simulink model "CT_SigmaDelta"  (Simulink 7.9)
settings: Solver=ode45  StartTime=0.0  StopTime=1  RelTol=1e-6
PreLoadFcn:
  | load one_stage.mat
libraries: dspmlti4 x7, simulink x2
(part 1 of 5)
settings Model: Creator=abehbood  LastModifiedBy=Arnaldi Isacco  CovSaveName=MOD  CovHTMLOptions=-sRT=1 -aTS=1 -bRG=1 -bTC=1 -hTR=0 -nFC=0 -scm=1 -bcm=1 -xEv=0  CovCumulativeVarName=MOD1
settings Model: CovPath=|
  | Averaging
  | Power Spectral
  | Density
settings SolverCC: ConsecutiveZCsStepRelTol=128*eps  ZeroCrossControl=DisableAll
settings DataIOCC: LimitDataPoints=off  SaveFormat=StructureWithTime  SaveOutput=off  SignalLogging=off  DSMLogging=off  SaveTime=off
settings OptimizationCC: InitFltsAndDblsToZero=on
settings DebuggingCC: AlgebraicLoopMsg=none  SaveWithParameterizedLinksMsg=none  SignalResolutionControl=TryResolveAllWithWarning  FcnCallInpInsideContextMsg=Use local settings  StrictBusMsg=Warning
settings SFSimCC: SimParseCustomCode=off
settings RTWCC: GenerateMakefile=off
settings GRTTargetCC: TargetFcnLib=ansi_tfl_tmw.mat  CombineOutputUpdateFcns=off  GRTInterface=on
settings ConfigurationSet: Description=SimMechanics 2G

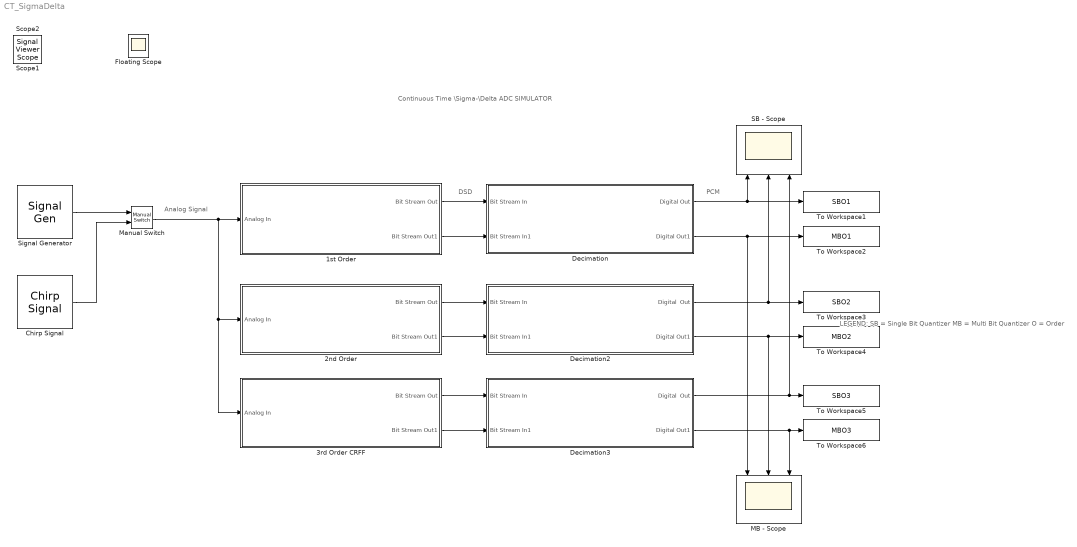
== system CT_SigmaDelta ==
  note: Continuous Time
      | \Sigma-\Delta ADC
      | SIMULATOR
  note: Analog Signal
  note: LEGEND:
      |
      | SB = Single Bit Quantizer
      |
      | MB = Multi Bit Quantizer
      |
      | O = Order
  note: DSD
  note: PCM
  1st Order : Subsystem
  "2nd Order  " : Subsystem
  3rd Order CRFF : Subsystem
  Chirp Signal : simulink/Sources/Chirp Signal  f1=0.1  T=24/24  f2=10000
  Decimation : Subsystem
  Decimation2 : Subsystem
  Decimation3 : Subsystem
  MB - Scope : Scope  NumInputPorts=3
      settings: ShowLegends=on  TimeRange=0.008  YMin=-1.25~-1.25~-1.25  YMax=1.25~1.25~1.25  SaveName=ScopeData2
  Manual Switch : simulink/Signal Routing/Manual Switch  sw=1  action=0  varsize=off
  SB - Scope : Scope  NumInputPorts=3
      settings: ShowLegends=on  TimeRange=0.008  YMin=-1.25~-1.25~-0.75  YMax=1.25~1.25~0.75
  Signal Generator : SignalGenerator  Frequency=6283  Units=rad/sec
  To Workspace1 : ToWorkspace  VariableName=SBO1  SampleTime=-1
  To Workspace2 : ToWorkspace  VariableName=MBO1  SampleTime=-1
  To Workspace3 : ToWorkspace  VariableName=SBO2  SampleTime=-1
  To Workspace4 : ToWorkspace  VariableName=MBO2  SampleTime=-1
  To Workspace5 : ToWorkspace  VariableName=SBO3  SampleTime=-1
  To Workspace6 : ToWorkspace  VariableName=MBO3  SampleTime=-1
  Floating Scope : Scope
      settings: Floating=on  YMin=-1  YMax=1
  Scope1 : SignalViewerScope  IOType=viewer  RefreshTime=0.035000
  Scope2 : SignalViewerScope  IOType=viewer  RefreshTime=0.035000
  wires:
  Decimation/1(Digital Out) -> SB - Scope/1, To Workspace1/1
  Decimation/2(Digital Out1) -> MB - Scope/1, To Workspace2/1
  Decimation2/1(Digital  Out) -> SB - Scope/2, To Workspace3/1
  Decimation2/2(Digital Out1) -> MB - Scope/2, To Workspace4/1
  Decimation3/1(Digital  Out) -> To Workspace5/1, SB - Scope/3
  Decimation3/2(Digital Out1) -> To Workspace6/1, MB - Scope/3
  1st Order/1(Bit Stream Out) -> Decimation/1(Bit Stream In)
  "2nd Order  "/1(Bit Stream Out) -> Decimation2/1(Bit Stream In)
  "2nd Order  "/2(Bit Stream Out1) -> Decimation2/2(Bit Stream In1)
  3rd Order CRFF/1(Bit Stream Out) -> Decimation3/1(Bit Stream In)
  3rd Order CRFF/2(Bit Stream Out1) -> Decimation3/2(Bit Stream In1)
  Signal Generator/1 -> Manual Switch/1
  Manual Switch/1 -> 1st Order/1("Analog In "), "2nd Order  "/1(Analog In), 3rd Order CRFF/1(Analog In)
  Chirp Signal/1 -> Manual Switch/2
  1st Order/2(Bit Stream Out1) -> Decimation/2(Bit Stream In1)

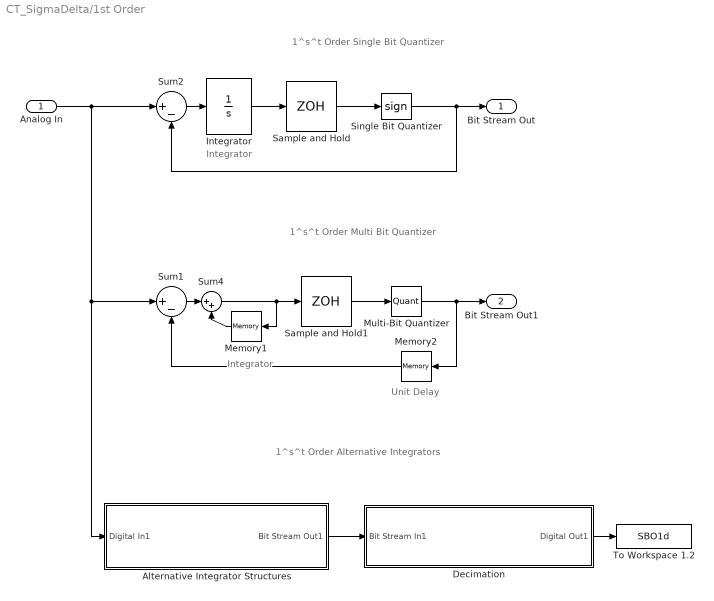
== system CT_SigmaDelta/1st Order ==
  note: 1^s^t Order Single Bit Quantizer
  note: 1^s^t Order Multi Bit Quantizer
  note: Integrator
  note: 1^s^t Order Alternative Integrators
  note: Unit Delay
  note: Integrator
  "Analog In " : Inport
  Alternative Integrator Structures : Subsystem
  Decimation : Subsystem
  Integrator : Integrator
  Memory1 : Memory  InheritSampleTime=on  LinearizeAsDelay=on
  Memory2 : Memory  InheritSampleTime=on  LinearizeAsDelay=on
  Multi-Bit Quantizer : Quantizer  QuantizationInterval=0.14  SampleTime=1/(48e3*64)
  Sample and Hold : ZeroOrderHold  SampleTime=1/(48e3*64)
  Sample and Hold1 : ZeroOrderHold  SampleTime=1/(48e3*64)
  Single Bit Quantizer : Signum  SampleTime=1/(48e3*64)
  Sum1 : Sum  Inputs=|+-  AccumDataTypeStr=double  SampleTime=1/(48e3*64)
  Sum2 : Sum  Inputs=|+-  AccumDataTypeStr=double  SampleTime=1/(48e3*64)
  Sum4 : Sum  Inputs=|++
  To Workspace 1.2 : ToWorkspace  VariableName=SBO1d  SampleTime=-1
  Bit Stream Out : Outport  OutDataTypeStr=double
  Bit Stream Out1 : Outport  Port=2  OutDataTypeStr=double
  wires:
  "Analog In "/1 -> Sum2/1, Sum1/1, Alternative Integrator Structures/1(Digital In1)
  Integrator/1 -> Sample and Hold/1
  Sum2/1 -> Integrator/1
  Sample and Hold/1 -> Single Bit Quantizer/1
  Single Bit Quantizer/1 -> Bit Stream Out/1, Sum2/2
  Alternative Integrator Structures/1(Bit Stream Out1) -> Decimation/1(Bit Stream In1)
  Decimation/1(Digital Out1) -> To Workspace 1.2/1
  Memory1/1 -> Sum4/2
  Sum4/1 -> Memory1/1, Sample and Hold1/1
  Sum1/1 -> Sum4/1
  Sample and Hold1/1 -> Multi-Bit Quantizer/1
  Multi-Bit Quantizer/1 -> Memory2/1, Bit Stream Out1/1
  Memory2/1 -> Sum1/2

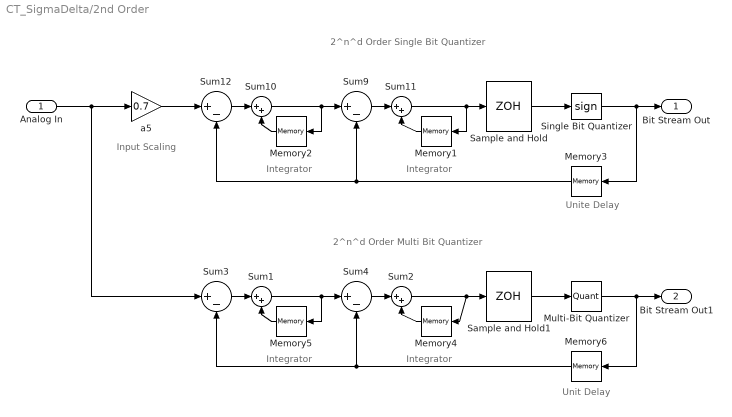
== system CT_SigmaDelta/2nd Order   ==
  note: 2^n^d Order Single Bit Quantizer
  note: 2^n^d Order Multi Bit Quantizer
  note: Input Scaling
  note: Integrator
  note: Integrator
  note: Integrator
  note: Integrator
  note: Unite Delay
  note: Unit Delay
  Analog In : Inport
  Memory{1..6} (6 alike) : Memory  InheritSampleTime=on  LinearizeAsDelay=on
  Multi-Bit Quantizer : Quantizer  QuantizationInterval=0.15  SampleTime=1/(48e3*64)
  Sample and Hold : ZeroOrderHold  SampleTime=1/(48e3*64)
  Sample and Hold1 : ZeroOrderHold  SampleTime=1/(48e3*64)
  Single Bit Quantizer : Signum  SampleTime=1/(48e3*64)
  Sum{1..2,10..11} (4 alike) : Sum  Inputs=|++  SampleTime=1/(48e3*64)
  Sum{3..4,9,12} (4 alike) : Sum  Inputs=|+-  AccumDataTypeStr=double  SampleTime=1/(48e3*64)
  a5 : Gain  Gain=0.7  SampleTime=1/(48e3*64)
  Bit Stream Out : Outport  OutDataTypeStr=double
  Bit Stream Out1 : Outport  Port=2  OutDataTypeStr=double
  wires:
  Analog In/1 -> a5/1, Sum3/1
  Sample and Hold/1 -> Single Bit Quantizer/1
  Sum9/1 -> Sum11/1
  Sum12/1 -> Sum10/1
  Single Bit Quantizer/1 -> Bit Stream Out/1, Memory3/1
  a5/1 -> Sum12/1
  Sample and Hold1/1 -> Multi-Bit Quantizer/1
  Sum4/1 -> Sum2/1
  Sum3/1 -> Sum1/1
  Multi-Bit Quantizer/1 -> Bit Stream Out1/1, Memory6/1
  Sum1/1 -> Sum4/1, Memory5/1
  Memory5/1 -> Sum1/2
  Sum10/1 -> Memory2/1, Sum9/1
  Memory2/1 -> Sum10/2
  Memory1/1 -> Sum11/2
  Sum11/1 -> Sample and Hold/1, Memory1/1
  Memory4/1 -> Sum2/2
  Sum2/1 -> Sample and Hold1/1, Memory4/1
  Memory3/1 -> Sum12/2, Sum9/2
  Memory6/1 -> Sum3/2, Sum4/2

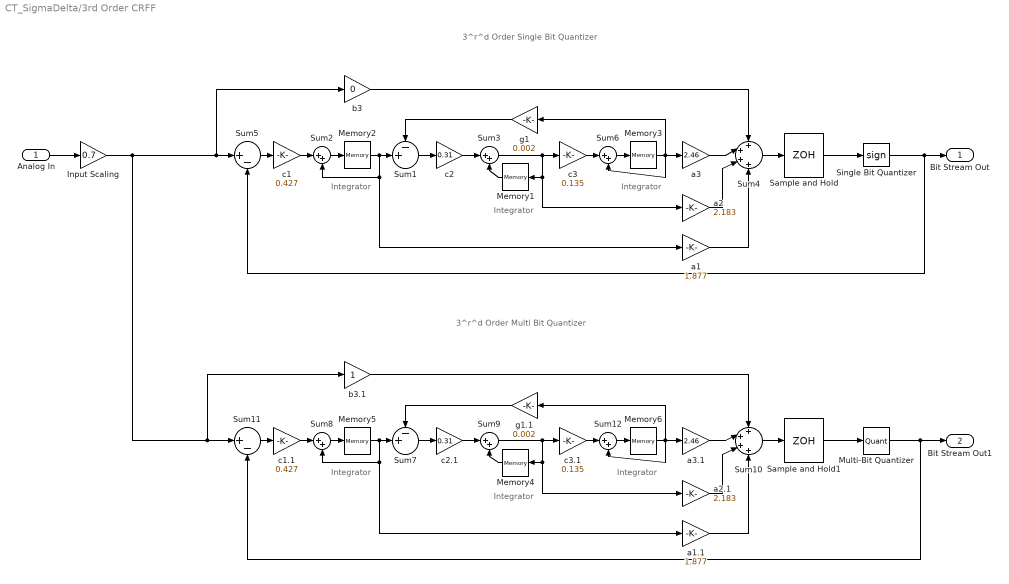
== system CT_SigmaDelta/3rd Order CRFF ==
  note: 3^r^d Order Single Bit Quantizer
  note: 3^r^d Order Multi Bit Quantizer
  note: Integrator
  note: Integrator
  note: Integrator
  note: Integrator
  note: Integrator
  note: Integrator
  Analog In : Inport
  Input Scaling : Gain  Gain=0.7  SampleTime=1/(48e3*64)
  Memory{1..6} (6 alike) : Memory  InheritSampleTime=on  LinearizeAsDelay=on
  Multi-Bit Quantizer : Quantizer  QuantizationInterval=0.125  SampleTime=1/(48e3*64)
  Sample and Hold : ZeroOrderHold  SampleTime=1/(48e3*64)
  Sample and Hold1 : ZeroOrderHold  SampleTime=1/(48e3*64)
  Single Bit Quantizer : Signum  SampleTime=1/(48e3*64)
  Sum1 : Sum  Inputs=-+|  AccumDataTypeStr=double  SampleTime=1/(48e3*64)
  Sum10 : Sum  Inputs=++++  AccumDataTypeStr=double  SampleTime=1/(48e3*64)
  Sum11 : Sum  Inputs=|+-  AccumDataTypeStr=double  SampleTime=1/(48e3*64)
  Sum{2..3,6,8..9,12} (6 alike) : Sum  Inputs=|++  SampleTime=1/(48e3*64)
  Sum4 : Sum  Inputs=++++  AccumDataTypeStr=double  SampleTime=1/(48e3*64)
  Sum5 : Sum  Inputs=|+-  AccumDataTypeStr=double  SampleTime=1/(48e3*64)
  Sum7 : Sum  Inputs=-+|  AccumDataTypeStr=double  SampleTime=1/(48e3*64)
  a1 : Gain  Gain=1.877  SampleTime=1/(48e3*64)
  a1.1 : Gain  Gain=1.877  SampleTime=1/(48e3*64)
  a2 : Gain  Gain=2.183  SampleTime=1/(48e3*64)
  a2.1 : Gain  Gain=2.183  SampleTime=1/(48e3*64)
  a3 : Gain  Gain=2.46  SampleTime=1/(48e3*64)
  a3.1 : Gain  Gain=2.46  SampleTime=1/(48e3*64)
  b3 : Gain  Gain=0  SampleTime=1/(48e3*64)
  b3.1 : Gain  SampleTime=1/(48e3*64)
  c1 : Gain  Gain=0.427  SampleTime=1/(48e3*64)
  c1.1 : Gain  Gain=0.427  SampleTime=1/(48e3*64)
  c2 : Gain  Gain=0.31  SampleTime=1/(48e3*64)
  c2.1 : Gain  Gain=0.31  SampleTime=1/(48e3*64)
  c3 : Gain  Gain=0.135  SampleTime=1/(48e3*64)
  c3.1 : Gain  Gain=0.135  SampleTime=1/(48e3*64)
  g1 : Gain  Gain=0.002  SampleTime=1/(48e3*64)
  g1.1 : Gain  Gain=0.002  SampleTime=1/(48e3*64)
  Bit Stream Out : Outport  OutDataTypeStr=double
  Bit Stream Out1 : Outport  Port=2  OutDataTypeStr=double
  wires:
  Analog In/1 -> Input Scaling/1
  Input Scaling/1 -> Sum5/1, b3/1, Sum11/1, b3.1/1
  a2/1 -> Sum4/3
  g1/1 -> Sum1/1
  Single Bit Quantizer/1 -> Sum5/2, Bit Stream Out/1
  Sum5/1 -> c1/1
  Sum1/1 -> c2/1
  c1/1 -> Sum2/1
  c2/1 -> Sum3/1
  c3/1 -> Sum6/1
  Memory1/1 -> Sum3/2
  Sum3/1 -> c3/1, Memory1/1, a2/1
  Sum4/1 -> Sample and Hold/1
  a1/1 -> Sum4/4
  a3/1 -> Sum4/2
  Sum2/1 -> Memory2/1
  Memory2/1 -> Sum1/2, Sum2/2, a1/1
  Sum6/1 -> Memory3/1
  Memory3/1 -> a3/1, Sum6/2, g1/1
  b3/1 -> Sum4/1
  Sample and Hold/1 -> Single Bit Quantizer/1
  a2.1/1 -> Sum10/3
  g1.1/1 -> Sum7/1
  Multi-Bit Quantizer/1 -> Bit Stream Out1/1, Sum11/2
  Sum11/1 -> c1.1/1
  Sum7/1 -> c2.1/1
  c1.1/1 -> Sum8/1
  c2.1/1 -> Sum9/1
  c3.1/1 -> Sum12/1
  Memory4/1 -> Sum9/2
  Sum9/1 -> a2.1/1, Memory4/1, c3.1/1
  Sum10/1 -> Sample and Hold1/1
  a1.1/1 -> Sum10/4
  a3.1/1 -> Sum10/2
  Sum8/1 -> Memory5/1
  Memory5/1 -> a1.1/1, Sum8/2, Sum7/2
  Sum12/1 -> Memory6/1
  Memory6/1 -> g1.1/1, Sum12/2, a3.1/1
  b3.1/1 -> Sum10/1
  Sample and Hold1/1 -> Multi-Bit Quantizer/1
